simulink model "modal_control_closed_loop_system"  (R2020b)
settings: Solver=VariableStepAuto  StartTime=0.0  StopTime=200  RelTol=1e-3
values from neighbouring files (symbols this model uses):
  COMMANDED_TORQUE_SATURATION = 0.05    [Workshop_MATLAB.m]
  COUPLING_COEFFICIENT = 0.5736    [Workshop_MATLAB.m]
  CUSTOM_POINTING_ERROR = 2.7*2*pi/360    (= 0.0471238898038)    [Workshop_MATLAB.m]
  DISTURBANCE_TORQUE = 0.001    [Workshop_MATLAB.m]
  DISTURBANCE_TORQUE_DELAY = 100    [Workshop_MATLAB.m]
  ESTIMATOR_TRANSFER_FUNCTION_DENOMINATOR = [ESTIMATOR_TIME_CONSTANT 1]    [Workshop_MATLAB.m]
  ESTIMATOR_TRANSFER_FUNCTION_NUMERATOR = [1 0]    [Workshop_MATLAB.m]
  feedForwardGain = gainMatrixStateFeedback(1)    [Workshop_MATLAB.m]
  FLEXIBLE_MODE_DAMPING_RATIO = 0.00495    [Workshop_MATLAB.m]
  FLEXIBLE_MODE_FREQUENCY = 2.6268    [Workshop_MATLAB.m]
  gainMatrixStateFeedback = generateModalControlGainMatrix(modalControlOpenLoop, targetDampingCoefficient, targetNaturalFrequency)    [Workshop_MATLAB.m]
  INITIAL_CONDITION_ON_STATE = 0.0001    [Workshop_MATLAB.m]
  LARGE_POINTING_ERROR = 10*2*pi/360    (= 0.174532925199)    [Workshop_MATLAB.m]
  MEASUREMENT_DELAY = 0.8    [Workshop_MATLAB.m]
  MEASUREMENT_NOISE_VARIANCE = 10^(-9)    (= 1e-09)    [Workshop_MATLAB.m]
  REACTION_WHEEL_DYNAMICS_DENOMINATOR = [1 2.400 0.763]    [Workshop_MATLAB.m]
  REACTION_WHEEL_DYNAMICS_NUMERATOR = REACTION_WHEEL_INERTIA*[1.214 0.763 0]    [Workshop_MATLAB.m]
  REACTION_WHEEL_INERTIA = 0.0004    [Workshop_MATLAB.m]
  REACTION_WHEEL_VELOCITY_SATURATION = 2800*2*pi/60    (= 293.215314335)    [Workshop_MATLAB.m]
  SATELLITE_INERTIA = 31.38    [Workshop_MATLAB.m]
  SMALL_POINTING_ERROR = 0.5*2*pi/360    (= 0.00872664625997)    [Workshop_MATLAB.m]
  STAR_TRACKER_NOISE_DELAY = 160    [Workshop_MATLAB.m]
settings Model: Creator=WLCG  LastModifiedBy=WLCG

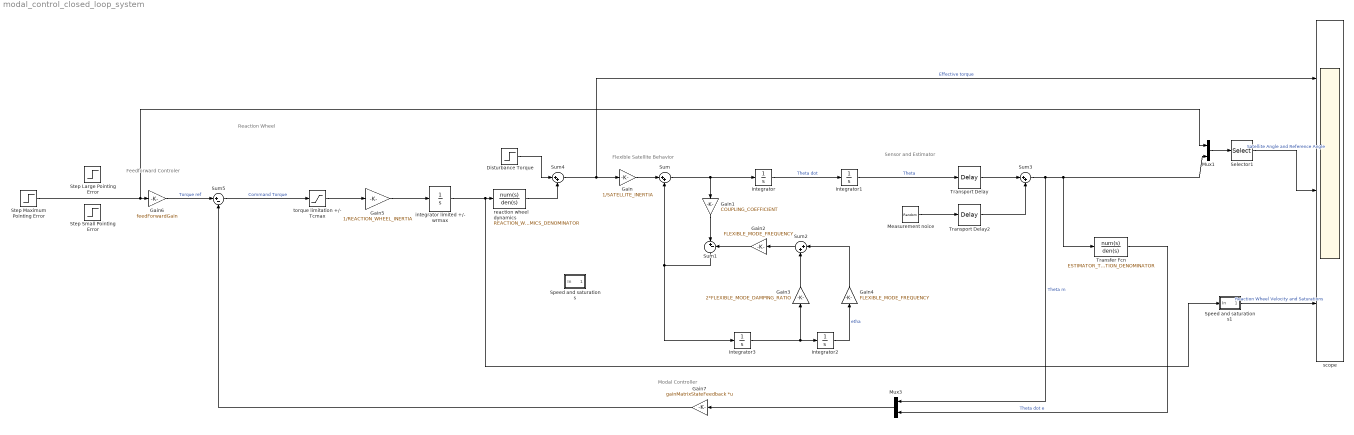
== system modal_control_closed_loop_system ==
  note: Modal Controller
  note: Feedforward Controler
  note: Sensor and Estimator
  note: Flexible Satellite Behavior
  note: Reaction Wheel
  Disturbance Torque : Step  Time=DISTURBANCE_TORQUE_DELAY  After=DISTURBANCE_TORQUE  SampleTime=0
  Gain : Gain  Gain=1/SATELLITE_INERTIA
  Gain1 : Gain  Gain=COUPLING_COEFFICIENT
  Gain2 : Gain  Gain=FLEXIBLE_MODE_FREQUENCY
  Gain3 : Gain  Gain=2*FLEXIBLE_MODE_DAMPING_RATIO
  Gain4 : Gain  Gain=FLEXIBLE_MODE_FREQUENCY
  Gain5 : Gain  Gain=1/REACTION_WHEEL_INERTIA
  Gain6 : Gain  Gain=feedForwardGain
  Gain7 : Gain  Gain=gainMatrixStateFeedback  Multiplication=Matrix(K*u) (u vector)
  Integrator : Integrator
  Integrator1 : Integrator
  Integrator2 : Integrator  InitialCondition=INITIAL_CONDITION_ON_STATE
  Integrator3 : Integrator
  Measurement noice : RandomNumber  Variance=MEASUREMENT_NOISE_VARIANCE  SampleTime=0.01
  Mux1 : Mux  Inputs=2
  Mux3 : Mux  Inputs=2
  Selector1 : Selector  InputPortWidth=2  IndexOptions=Index vector (dialog)  Indices=[2 1]  OutputSizes=1
  Speed and saturations : Subsystem
  Speed and saturations1 : Subsystem
  Step Large Pointing Error : Step  Time=0  After=LARGE_POINTING_ERROR  SampleTime=0
  Step Maximum Pointing Error : Step  Time=0  After=CUSTOM_POINTING_ERROR  SampleTime=0
  Step Small Pointing Error : Step  Time=0  After=SMALL_POINTING_ERROR  SampleTime=0
  Sum{,2..4} (4 alike) : Sum  Inputs=|++
  Sum1 : Sum  Inputs=|+-
  Sum5 : Sum  Inputs=|+-
  Transfer Fcn : TransferFcn  Numerator=ESTIMATOR_TRANSFER_FUNCTION_NUMERATOR  Denominator=ESTIMATOR_TRANSFER_FUNCTION_DENOMINATOR
  Transport Delay : TransportDelay  DelayTime=MEASUREMENT_DELAY
  Transport Delay2 : TransportDelay  DelayTime=STAR_TRACKER_NOISE_DELAY
  integrator limited +/- wrmax : Integrator  LimitOutput=on  UpperSaturationLimit=REACTION_WHEEL_VELOCITY_SATURATION  LowerSaturationLimit=-REACTION_WHEEL_VELOCITY_SATURATION
  reaction wheel dynamics : TransferFcn  Numerator=REACTION_WHEEL_DYNAMICS_NUMERATOR  Denominator=REACTION_WHEEL_DYNAMICS_DENOMINATOR
  scope : Scope  NumInputPorts=3
  torque limitation +/- Tcmax : Saturate  UpperLimit=COMMANDED_TORQUE_SATURATION  LowerLimit=-COMMANDED_TORQUE_SATURATION
  wires:
  Integrator2/1 -> Gain4/1  "etha"
  Gain4/1 -> Sum2/1
  Gain3/1 -> Sum2/2
  Sum/1 -> Gain1/1, Integrator/1
  Sum5/1 -> torque limitation +/- Tcmax/1  "Command Torque"
  Sum1/1 -> Sum/2, Integrator3/1
  Integrator3/1 -> Integrator2/1, Gain3/1
  Gain2/1 -> Sum1/2
  Sum2/1 -> Gain2/1
  Gain/1 -> Sum/1
  Gain1/1 -> Sum1/1
  Integrator/1 -> Integrator1/1  "Theta dot"
  torque limitation +/- Tcmax/1 -> Gain5/1
  integrator limited +/- wrmax/1 -> Speed and saturations1/1(In), reaction wheel dynamics/1
  Gain5/1 -> integrator limited +/- wrmax/1
  Sum3/1 -> Mux3/1, Mux1/2, Transfer Fcn/1  "Theta m"
  Transport Delay/1 -> Sum3/1
  Measurement noice/1 -> Transport Delay2/1
  Transfer Fcn/1 -> Mux3/2  "Theta dot e"
  reaction wheel dynamics/1 -> Sum4/2
  Integrator1/1 -> Transport Delay/1  "Theta"
  Sum4/1 -> scope/1, Gain/1  "Effective torque"
  Disturbance Torque/1 -> Sum4/1
  Transport Delay2/1 -> Sum3/2
  Mux1/1 -> Selector1/1
  Selector1/1 -> scope/2  "Satellite Angle and Reference Angle"
  Gain6/1 -> Sum5/1  "Torque ref"
  Gain7/1 -> Sum5/2
  Mux3/1 -> Gain7/1
  Step Maximum Pointing Error/1 -> Mux1/1, Gain6/1
  Speed and saturations1/1(Mux) -> scope/3  "Reaction Wheel Velocity and Saturations"

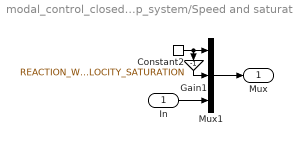
== system modal_control_closed_loop_system/Speed and saturations ==
  In : Inport
  Constant2 : Constant  Value=REACTION_WHEEL_VELOCITY_SATURATION
  Gain1 : Gain  Gain=-1
  Mux1 : Mux  Inputs=3
  Mux : Outport
  wires:
  Gain1/1 -> Mux1/2
  In/1 -> Mux1/3
  Mux1/1 -> Mux/1
  Constant2/1 -> Gain1/1, Mux1/1

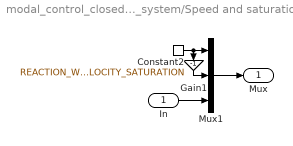
== system modal_control_closed_loop_system/Speed and saturations1 ==
  In : Inport
  Constant2 : Constant  Value=REACTION_WHEEL_VELOCITY_SATURATION
  Gain1 : Gain  Gain=-1
  Mux1 : Mux  Inputs=3
  Mux : Outport
  wires:
  Gain1/1 -> Mux1/2
  In/1 -> Mux1/3
  Mux1/1 -> Mux/1
  Constant2/1 -> Gain1/1, Mux1/1
